simulink library "ESys"  (R2025a)
settings: Solver=VariableStepAuto  StartTime=0.0  StopTime=10.0  RelTol=1e-3
undefined symbols (not defined in the file): bm, Jm, Ki, Kp, Kphi, La, N, Ra, Ts_PID, TTL_amplitude, TTL_on, Va_batt, w_max
libraries: $bdroot x3, simulink x2, slpidlib x1, eePwmGenerator x1
settings Model: Creator=tecnicomcbti  LastModifiedBy=mcbti_speedgoat

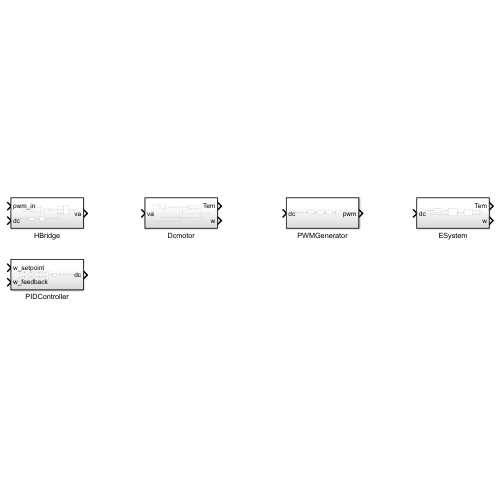
[thumbnail: Simulink's stored preview of the top-level diagram]
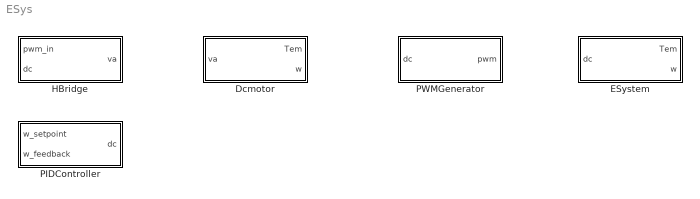
== system ESys ==
  Dcmotor : Subsystem
  ESystem : Subsystem
  HBridge : Subsystem
  PIDController : Subsystem
  PWMGenerator : Subsystem

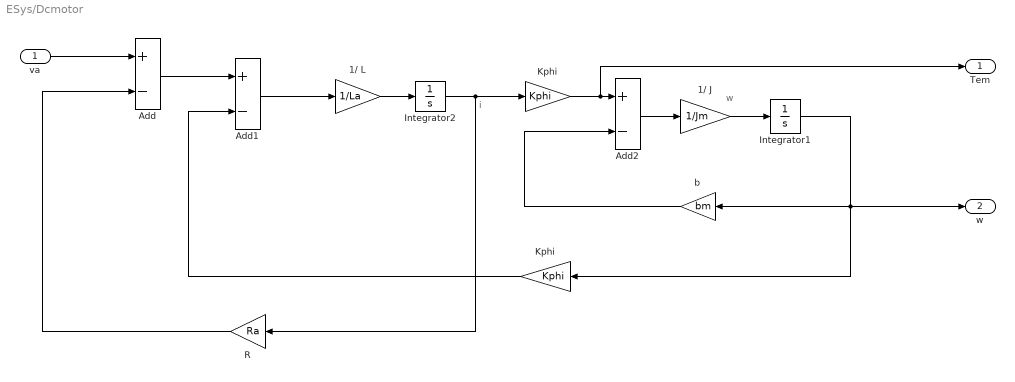
== system ESys/Dcmotor ==
  note: i
  note: w
  va : Inport
  1/ J : Gain  Gain=1/Jm
  1/ L : Gain  Gain=1/La
  Add : Sum  Inputs=+-
  Add1 : Sum  Inputs=+-
  Add2 : Sum  Inputs=+-
  Integrator1 : Integrator
  Integrator2 : Integrator
  Kphi : Gain  Gain=Kphi
  "Kphi " : Gain  Gain=Kphi
  R : Gain  Gain=Ra
  b : Gain  Gain=bm
  Tem : Outport
  w : Outport  Port=2
  wires:
  Kphi/1 -> Tem/1, Add2/1
  Integrator2/1 -> R/1, Kphi/1
  Add1/1 -> 1/ L/1
  Add2/1 -> 1/ J/1
  va/1 -> Add/1
  b/1 -> Add2/2
  R/1 -> Add/2
  1/ J/1 -> Integrator1/1
  "Kphi "/1 -> Add1/2
  1/ L/1 -> Integrator2/1
  Integrator1/1 -> w/1, "Kphi "/1, b/1
  Add/1 -> Add1/1

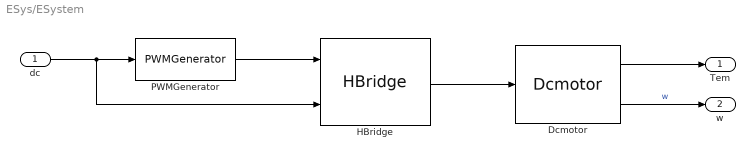
== system ESys/ESystem ==
  dc : Inport
  Dcmotor : $bdroot/Dcmotor  SystemSampleTime=-1  VariantActivationTime=update diagram  EmptyChoice=off  PassThrough=off  PassThroughVariantControl=(default)  EmptyChoiceVariantControl=(default)  AllowFlexibleInterface=on  Latency=0  AutoFrameSizeCalculation=off
  HBridge : $bdroot/HBridge  SystemSampleTime=-1  VariantActivationTime=update diagram  EmptyChoice=off  PassThrough=off  PassThroughVariantControl=(default)  EmptyChoiceVariantControl=(default)  AllowFlexibleInterface=on  Latency=0  AutoFrameSizeCalculation=off
  PWMGenerator : $bdroot/PWMGenerator  SystemSampleTime=-1  VariantActivationTime=update diagram  EmptyChoice=off  PassThrough=off  PassThroughVariantControl=(default)  EmptyChoiceVariantControl=(default)  AllowFlexibleInterface=on  Latency=0  AutoFrameSizeCalculation=off
  Tem : Outport
  w : Outport  Port=2
  wires:
  PWMGenerator/1 -> HBridge/1
  HBridge/1 -> Dcmotor/1
  dc/1 -> HBridge/2, PWMGenerator/1
  Dcmotor/1 -> Tem/1
  Dcmotor/2 -> w/1  "w"

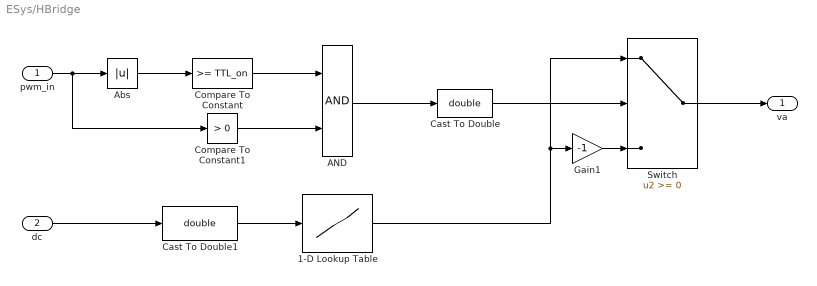
== system ESys/HBridge ==
  pwm_in : Inport
  dc : Inport  Port=2
  1-D Lookup Table : Lookup_n-D  NumberOfTableDimensions=1  BreakpointsForDimension1=double(linspace(0,1,20))  Table=double(Va_batt.*linspace(0,1,20))  ExtrapMethod=Clip  InternalRulePriority=Speed  RndMeth=Simplest
  AND : Logic  AllPortsSameDT=off  OutDataTypeStr=boolean
  Abs : Abs  SaturateOnIntegerOverflow=off
  Cast To Double : DataTypeConversion  OutDataTypeStr=double  SaturateOnIntegerOverflow=off  RndMeth=Floor
  Cast To Double1 : DataTypeConversion  OutDataTypeStr=double  SaturateOnIntegerOverflow=off  RndMeth=Floor
  Compare To Constant : simulink/Logic and Bit Operations/Compare To Constant  relop=>=  const=TTL_on  OutDataTypeStr=boolean
  Compare To Constant1 : simulink/Logic and Bit Operations/Compare To Constant  relop=>  const=0  OutDataTypeStr=boolean
  Gain1 : Gain  Gain=-1
  Switch : Switch  SaturateOnIntegerOverflow=off  InputSameDT=off
  va : Outport
  wires:
  1-D Lookup Table/1 -> Switch/1, Gain1/1
  dc/1 -> Cast To Double1/1
  Switch/1 -> va/1
  Gain1/1 -> Switch/3
  Cast To Double/1 -> Switch/2
  Compare To Constant/1 -> AND/1
  pwm_in/1 -> Compare To Constant1/1, Abs/1
  AND/1 -> Cast To Double/1
  Compare To Constant1/1 -> AND/2
  Cast To Double1/1 -> 1-D Lookup Table/1
  Abs/1 -> Compare To Constant/1

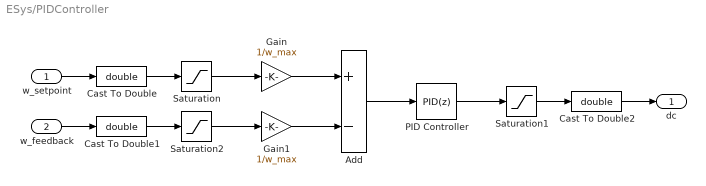
== system ESys/PIDController ==
  w_setpoint : Inport
  w_feedback : Inport  Port=2
  Add : Sum  Inputs=+-
  Cast To Double : DataTypeConversion  OutDataTypeStr=double  SaturateOnIntegerOverflow=off  RndMeth=Floor
  Cast To Double1 : DataTypeConversion  OutDataTypeStr=double  SaturateOnIntegerOverflow=off  RndMeth=Floor
  Cast To Double2 : DataTypeConversion  OutDataTypeStr=double  SaturateOnIntegerOverflow=off  RndMeth=Floor
  Gain : Gain  Gain=1/w_max
  Gain1 : Gain  Gain=1/w_max
  PID Controller : slpidlib/PID Controller  Controller=PID  Form=Parallel  TimeDomain=Discrete-time  UseExternalTs=off  SampleTime=Ts_PID  IntegratorMethod=Forward Euler  FilterMethod=Forward Euler  ControllerParametersSource=internal  P=Kp  I=Ki  UseKiTs=off  D=0  UseExternalDerivativeSource=off  N=N  UseFilter=on  TunerSelectOption=Transfer Function Based (PID Tuner App)  InitialConditionSource=internal  InitialConditionForIntegrator=0  InitialConditionForFilter=0  DifferentiatorICPrevScaledInput=0  ExternalReset=none  TrackingMode=off  Kt=1  LimitOutput=off  SatLimitsSource=internal  UpperSaturationLimit=inf  LowerSaturationLimit=-inf  LinearizeAsGain=on  AntiWindupMode=none  Kb=1  LimitIntegrator=off  UpperIntegratorSaturationLimit=inf  LowerIntegratorSaturationLimit=-inf  POutMin=[]  POutMax=[]  IOutMin=[]  IOutMax=[]  DOutMin=[]  DOutMax=[]  NOutMin=[]  NOutMax=[]  SumOutMin=[]  SumOutMax=[]  SaturationOutMin=[]  SaturationOutMax=[]  PParamMin=[]  PParamMax=[]  IParamMin=[]  IParamMax=[]  DParamMin=[]  DParamMax=[]  NParamMin=[]  NParamMax=[]  KbParamMin=[]  KbParamMax=[]  KtParamMin=[]  KtParamMax=[]  KbOutMin=[]  KbOutMax=[]  KtOutMin=[]  KtOutMax=[]  IntegratorOutMin=[]  IntegratorOutMax=[]  FilterOutMin=[]  FilterOutMax=[]  SumI1OutMin=[]  SumI1OutMax=[]  SumI2OutMin=[]  SumI2OutMax=[]  SumI3OutMin=[]  SumI3OutMax=[]  SumI4OutMin=[]  SumI4OutMax=[]  SumDOutMin=[]  SumDOutMax=[]  DifferentiatorOutMin=[]  DifferentiatorOutMax=[]  FilterDiffOutCoefMin=[]  FilterDiffOutCoefMax=[]  ReciprocalOutMin=[]  ReciprocalOutMax=[]  SumDenOutMin=[]  SumDenOutMax=[]  SumNumOutMin=[]  SumNumOutMax=[]  DivideOutMin=[]  DivideOutMax=[]  UdiffTsProdOutMin=[]  UdiffTsProdOutMax=[]  NTsProdOutMin=[]  NTsProdOutMax=[]  UintegralTsProdOutMin=[]  UintegralTsProdOutMax=[]  UngainTsProdOutMin=[]  UngainTsProdOutMax=[]  ClampingZeroOutDataTypeStr=Inherit: Inherit via back propagation  ClampingZeroOutMin=[]  ClampingZeroOutMax=[]  FilterDenConstantOutDataTypeStr=Inherit: Inherit via back propagation  FilterDenConstantOutMin=[]  FilterDenConstantOutMax=[]  PCopyOutDataTypeStr=Inherit: Inherit via back propagation  PCopyOutMin=[]  PCopyOutMax=[]  NCopyOutDataTypeStr=Inherit: Inherit via back propagation  NCopyOutMin=[]  NCopyOutMax=[]  IntegratorContinuousStateAttributes=''  IntegratorStateMustResolveToSignalObject=off  IntegratorRTWStateStorageClass=Auto  FilterContinuousStateAttributes=''  FilterStateMustResolveToSignalObject=off  FilterRTWStateStorageClass=Auto  ParallelPVariant=InternalParameters  IdealPVariant=Disabled  IVariant=InternalParameters  DVariant=InternalParameters  IntegratorVariant=Discrete  SatVariant=Disabled  AWVariant=Passthrough  PCopyVariant=Disabled  TRVariant=Disabled  FdbkBlocksVariant=Forward  IdealPFdbkVariant=Disabled  SatFdbkVariant=Disabled  DerivativeFilterVariant=ForwardEulerFilter  NVariant=InternalParameters  NCopyVariant=Disabled  FilterICVariant=InternalICsFilter  IntegratorICVariant=InternalICs  ExternalResetVariant=Disabled  TRSumVariant=Passthrough  SumFdbkVariant=Disabled  SumVariant=Sum_PID  TsampFilterVariant=InternalTs  TsampNgainVariant=Passthrough  TsampIntegralVariant=Disabled_SignalSpec  ExternalSaturationOutDataTypeStr=Inherit: Same as second input  DerivativeSourceVariant=ErrorSignal  PreIntVariant=InternalPreInt
  Saturation : Saturate  UpperLimit=w_max  LowerLimit=0
  Saturation1 : Saturate  UpperLimit=1  LowerLimit=0
  Saturation2 : Saturate  UpperLimit=w_max  LowerLimit=0
  dc : Outport
  wires:
  w_setpoint/1 -> Cast To Double/1
  w_feedback/1 -> Cast To Double1/1
  Cast To Double2/1 -> dc/1
  Gain/1 -> Add/1
  Cast To Double1/1 -> Saturation2/1
  Cast To Double/1 -> Saturation/1
  Saturation/1 -> Gain/1
  Gain1/1 -> Add/2
  Saturation2/1 -> Gain1/1
  Add/1 -> PID Controller/1
  Saturation1/1 -> Cast To Double2/1
  PID Controller/1 -> Saturation1/1

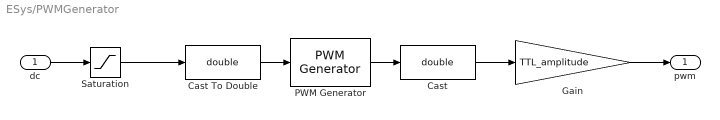
== system ESys/PWMGenerator ==
  dc : Inport
  Cast : DataTypeConversion  OutDataTypeStr=double  SaturateOnIntegerOverflow=off  RndMeth=Floor
  Cast To Double : DataTypeConversion  OutDataTypeStr=double  SaturateOnIntegerOverflow=off  RndMeth=Floor
  Gain : Gain  Gain=TTL_amplitude
  PWM Generator : eePwmGenerator/PWM Generator  CarrCount=Up  Tper=0.001  Tdelay=0  Ts=1e-4
  Saturation : Saturate  UpperLimit=1  LowerLimit=0
  pwm : Outport
  wires:
  dc/1 -> Saturation/1
  Saturation/1 -> Cast To Double/1
  Cast/1 -> Gain/1
  Gain/1 -> pwm/1
  Cast To Double/1 -> PWM Generator/1
  PWM Generator/1 -> Cast/1
